simulink model "PreBraking_Scenario2_cs"  (R2014b)
settings: Solver=ode5  SolverMode=SingleTasking  StartTime=0.0  StopTime=inf  FixedStep=1/100  RelTol=1e-3
PreLoadFcn:
  | mbxruntime.callbacks.PreLoadFcn(bdroot);
  | check_NUTS_defined;
  | 
  | assignin('base',['model_closed_' bdroot],false);addpath('../includes_AEBS');
PostLoadFcn:
  | mbxruntime.callbacks.PostLoadFcn(bdroot);
InitFcn:
  | mbxruntime.callbacks.InitFcn(bdroot);
StartFcn:
  | mbxruntime.callbacks.StartFcn(bdroot);
StopFcn:
  | mbxruntime.callbacks.StopFcn(bdroot);
model workspace: external: MAT-File .\PreBraking_Scenario2_cs_hws.mat (data not in the file)
undefined symbols (not defined in the file or in its folder): mbxruntime, OrientationPitch, OrientationRoll, PositionX, PositionY, PositionZ, tabledata, warningInitialVelocity, x0
undefined symbols (not defined in the file): PreBraking_Scenario2_cs_03ca8bbbeab2b9b9, PreBraking_Scenario2_cs_060f8d532884bc4b, PreBraking_Scenario2_cs_06c37d8c8719462d, PreBraking_Scenario2_cs_0d3de4e10595602b, PreBraking_Scenario2_cs_132afc293d4bc970, PreBraking_Scenario2_cs_135fb3525bf57813, PreBraking_Scenario2_cs_199db523920b0ae8, PreBraking_Scenario2_cs_19b5c7fc995ca371, PreBraking_Scenario2_cs_1c0d05c0e95fb3bc, PreBraking_Scenario2_cs_230ed70c3742a1eb, PreBraking_Scenario2_cs_2a9a795ed7b4eca0, PreBraking_Scenario2_cs_2aad3e26cef81116, PreBraking_Scenario2_cs_3112792458948f16, PreBraking_Scenario2_cs_31511e5cf664957f, PreBraking_Scenario2_cs_335bc07f9f9d6bb2, PreBraking_Scenario2_cs_343e102d67d9e47c, PreBraking_Scenario2_cs_38754ff77a13247b, PreBraking_Scenario2_cs_3f42c52076d9af39, PreBraking_Scenario2_cs_4b3e07bd10cdcbdf, PreBraking_Scenario2_cs_4d97be448e41c5e7, PreBraking_Scenario2_cs_50fbc7e9b9a11bbd, PreBraking_Scenario2_cs_54739860340bd271, PreBraking_Scenario2_cs_5a356ab1c62c8f7e, PreBraking_Scenario2_cs_5b4437f6719e0d1b, PreBraking_Scenario2_cs_5c234b912a76c6a5, PreBraking_Scenario2_cs_6168355cd5f7aa5b, PreBraking_Scenario2_cs_622a303a40218b4d, PreBraking_Scenario2_cs_647713569694f0a8, PreBraking_Scenario2_cs_69cfdaef90de11b6, PreBraking_Scenario2_cs_6af59d93ed31b258, PreBraking_Scenario2_cs_6b0b2c155afad700, PreBraking_Scenario2_cs_6b0e277e7fb709ae, PreBraking_Scenario2_cs_6cdb8944f433c9b5, PreBraking_Scenario2_cs_6e61e0d6d53946a8, PreBraking_Scenario2_cs_721bd4ea87d705e5, PreBraking_Scenario2_cs_733181add4a3a2bd, PreBraking_Scenario2_cs_7a4dfa61d77329b3, PreBraking_Scenario2_cs_7b6eba6e821515af, PreBraking_Scenario2_cs_7dfcf0aa2939e252, PreBraking_Scenario2_cs_7f39d304a27b340b, PreBraking_Scenario2_cs_8077b8dca741d53f, PreBraking_Scenario2_cs_83874eeccd6bc572, PreBraking_Scenario2_cs_8e3f6b53dcde3bb3, PreBraking_Scenario2_cs_98c5cdaae36d0717, PreBraking_Scenario2_cs_98cfc98f5f5b01fc, PreBraking_Scenario2_cs_9906f28f708d2a62, PreBraking_Scenario2_cs_a13988e047af266f, PreBraking_Scenario2_cs_a8fd4bfaed66c690, PreBraking_Scenario2_cs_a93f6bf774ad8002, PreBraking_Scenario2_cs_a9ad9a9d247ad05d, PreBraking_Scenario2_cs_ab408108b3f0fc97, PreBraking_Scenario2_cs_Audi_A8_3_Dynamics_Simple_initialPitch, PreBraking_Scenario2_cs_Audi_A8_3_Dynamics_Simple_initialRoll, PreBraking_Scenario2_cs_Audi_A8_3_Dynamics_Simple_initialX, PreBraking_Scenario2_cs_Audi_A8_3_Dynamics_Simple_initialY, PreBraking_Scenario2_cs_Audi_A8_3_Dynamics_Simple_initialYaw, PreBraking_Scenario2_cs_Audi_A8_3_Dynamics_Simple_initialZ, PreBraking_Scenario2_cs_b1fc7fed98e6f1a7, PreBraking_Scenario2_cs_b75ef87da1419b4e, PreBraking_Scenario2_cs_b7a6524fab202de5 ... (+41)
libraries: simulink_extras x81, PreScanSimulinkLibrary x27, simulink x20, PreScanUsefulBlocks x2
(part 29 of 33)

== system PreBraking_Scenario2_cs/WheelL0_Citroen_C3_2/Actuator/visu_Rotate ==
  In1 : Inport
  sfun_RPYActuator : S-Function  FunctionName=sfun_RPYActuator  Parameters=SParameter1, SParameter2, SampleTime  EnableBusSupport=off  mask(Legacy Function){SFunctionSpec=void prescan_outputFcn(void ** work1,  PRESCAN_XYZ_DATA u1[1]), SParameter1=UniqueID, SParameter2=uint8([Object3DID 0]), SampleTime=TimeStep, ShowSpec=on}
      mask prompts: SParameter1 "P1:"; SParameter2 "P2:"; SampleTime "Sample time (-1 for inherited):"; ShowSpec "Display function specification"
      mask help:
      | This block allows you to call the legacy functions specified by the following Legacy Code Tool definition:
      | def.SFunctionName = 'sfun_PositionActuator';
      | def.OutputFcnSpec = 'void prescan_outputFcn(void ** work1,  PRESCAN_XYZ_DATA u1[1])';
      | def.StartFcnSpec = 'void prescan_startFcn(void ** work1, uint8 p1[], double p2)';
      | def.TerminateFcnSpec = 'void prescan_terminateFcn(void ** work1)';
      | def.HeaderFiles = {'prescan_positionactuator_data.h', 'prescan_header_data.h', 'prescan_SFunLibrary.h', 'prescan_CreateLogHandler.h', 'prescan_CreateErrorHandler.h'};
      | def.SourceFiles = {'prescan_MexLogHandler.cpp', 'prescan_SimStructErrorHandler.cpp', 'prescan_ConcurrentLogHandler.cpp', 'prescan_ConcurrentErrorHandler.cpp'};
      | def.HostLibFiles = {'sensorinterfaced.lib'};
      | def.TargetLibFiles = {'sensorinterfaced.so'};
      | def.IncPaths = {'.', 'C:\prescandev\vislibrary\vis\..\pimp\include\sensors\InterfaceRTW'};
      | def.SrcPaths = {'.'};
      | def.LibPaths = {'C:\\prescandev\\vislibrary_build\lib'};
      | def.SampleTime = 'parameterized';
      mask Help: <p>This block was generated automatically by the Legacy Code Tool. For detailed help on this tool, call<a href="matlab:legacy_code('help')"> legacy_code('help')</a>.</p>
      mask Callback ShowSpec:
      | if strcmp(get_param(gcbh, 'ShowSpec'), 'on')
      |   set_param(gcbh, 'MaskDisplay', sprintf('fprintf(''%s'');', get_param(gcbh, 'SFunctionSpec')));
      | else
      |   set_param(gcbh, 'MaskDisplay', sprintf('fprintf(''%s'');', get_param(gcbh, 'FunctionName')));
      | end
      mask Display: fprintf('void prescan_outputFcn(void ** work1,  PRESCAN_RPY_DATA u1[1])');
  wires:
  In1/1 -> sfun_RPYActuator/1

== system PreBraking_Scenario2_cs/WheelL0_Citroen_C3_2/Actuator/visu_Translate ==
  In1 : Inport
  sfun_PositionActuator : S-Function  FunctionName=sfun_PositionActuator  Parameters=SParameter1, SParameter2, SampleTime  EnableBusSupport=off  mask(Legacy Function){SFunctionSpec=void prescan_outputFcn(void ** work1,  PRESCAN_XYZ_DATA u1[1]), SParameter1=uint8([Object3DID 0]), SParameter2=UniqueID, SampleTime=TimeStep, ShowSpec=on}
      mask prompts: SParameter1 "P1:"; SParameter2 "P2:"; SampleTime "Sample time (-1 for inherited):"; ShowSpec "Display function specification"
      mask help:
      | This block allows you to call the legacy functions specified by the following Legacy Code Tool definition:
      | def.SFunctionName = 'sfun_PositionActuator';
      | def.OutputFcnSpec = 'void prescan_outputFcn(void ** work1,  PRESCAN_XYZ_DATA u1[1])';
      | def.StartFcnSpec = 'void prescan_startFcn(void ** work1, uint8 p1[], double p2)';
      | def.TerminateFcnSpec = 'void prescan_terminateFcn(void ** work1)';
      | def.HeaderFiles = {'prescan_positionactuator_data.h', 'prescan_header_data.h', 'prescan_SFunLibrary.h', 'prescan_CreateLogHandler.h', 'prescan_CreateErrorHandler.h'};
      | def.SourceFiles = {'prescan_MexLogHandler.cpp', 'prescan_SimStructErrorHandler.cpp', 'prescan_ConcurrentLogHandler.cpp', 'prescan_ConcurrentErrorHandler.cpp'};
      | def.HostLibFiles = {'sensorinterfaced.lib'};
      | def.TargetLibFiles = {'sensorinterfaced.so'};
      | def.IncPaths = {'.', 'C:\prescandev\vislibrary\vis\..\pimp\include\sensors\InterfaceRTW'};
      | def.SrcPaths = {'.'};
      | def.LibPaths = {'C:\\prescandev\\vislibrary_build\lib'};
      | def.SampleTime = 'parameterized';
      mask Help: <p>This block was generated automatically by the Legacy Code Tool. For detailed help on this tool, call<a href="matlab:legacy_code('help')"> legacy_code('help')</a>.</p>
      mask Callback ShowSpec:
      | if strcmp(get_param(gcbh, 'ShowSpec'), 'on')
      |   set_param(gcbh, 'MaskDisplay', sprintf('fprintf(''%s'');', get_param(gcbh, 'SFunctionSpec')));
      | else
      |   set_param(gcbh, 'MaskDisplay', sprintf('fprintf(''%s'');', get_param(gcbh, 'FunctionName')));
      | end
      mask Display: fprintf('void prescan_outputFcn(void ** work1,  PRESCAN_XYZ_DATA u1[1])');
  wires:
  In1/1 -> sfun_PositionActuator/1

== system PreBraking_Scenario2_cs/WheelL0_Fiat_Bravo_2/Actuator/visu_Rotate ==
  In1 : Inport
  sfun_RPYActuator : S-Function  FunctionName=sfun_RPYActuator  Parameters=SParameter1, SParameter2, SampleTime  EnableBusSupport=off  mask(Legacy Function){SFunctionSpec=void prescan_outputFcn(void ** work1,  PRESCAN_XYZ_DATA u1[1]), SParameter1=UniqueID, SParameter2=uint8([Object3DID 0]), SampleTime=TimeStep, ShowSpec=on}
      mask prompts: SParameter1 "P1:"; SParameter2 "P2:"; SampleTime "Sample time (-1 for inherited):"; ShowSpec "Display function specification"
      mask help:
      | This block allows you to call the legacy functions specified by the following Legacy Code Tool definition:
      | def.SFunctionName = 'sfun_PositionActuator';
      | def.OutputFcnSpec = 'void prescan_outputFcn(void ** work1,  PRESCAN_XYZ_DATA u1[1])';
      | def.StartFcnSpec = 'void prescan_startFcn(void ** work1, uint8 p1[], double p2)';
      | def.TerminateFcnSpec = 'void prescan_terminateFcn(void ** work1)';
      | def.HeaderFiles = {'prescan_positionactuator_data.h', 'prescan_header_data.h', 'prescan_SFunLibrary.h', 'prescan_CreateLogHandler.h', 'prescan_CreateErrorHandler.h'};
      | def.SourceFiles = {'prescan_MexLogHandler.cpp', 'prescan_SimStructErrorHandler.cpp', 'prescan_ConcurrentLogHandler.cpp', 'prescan_ConcurrentErrorHandler.cpp'};
      | def.HostLibFiles = {'sensorinterfaced.lib'};
      | def.TargetLibFiles = {'sensorinterfaced.so'};
      | def.IncPaths = {'.', 'C:\prescandev\vislibrary\vis\..\pimp\include\sensors\InterfaceRTW'};
      | def.SrcPaths = {'.'};
      | def.LibPaths = {'C:\\prescandev\\vislibrary_build\lib'};
      | def.SampleTime = 'parameterized';
      mask Help: <p>This block was generated automatically by the Legacy Code Tool. For detailed help on this tool, call<a href="matlab:legacy_code('help')"> legacy_code('help')</a>.</p>
      mask Callback ShowSpec:
      | if strcmp(get_param(gcbh, 'ShowSpec'), 'on')
      |   set_param(gcbh, 'MaskDisplay', sprintf('fprintf(''%s'');', get_param(gcbh, 'SFunctionSpec')));
      | else
      |   set_param(gcbh, 'MaskDisplay', sprintf('fprintf(''%s'');', get_param(gcbh, 'FunctionName')));
      | end
      mask Display: fprintf('void prescan_outputFcn(void ** work1,  PRESCAN_RPY_DATA u1[1])');
  wires:
  In1/1 -> sfun_RPYActuator/1

== system PreBraking_Scenario2_cs/WheelL0_Fiat_Bravo_2/Actuator/visu_Translate ==
  In1 : Inport
  sfun_PositionActuator : S-Function  FunctionName=sfun_PositionActuator  Parameters=SParameter1, SParameter2, SampleTime  EnableBusSupport=off  mask(Legacy Function){SFunctionSpec=void prescan_outputFcn(void ** work1,  PRESCAN_XYZ_DATA u1[1]), SParameter1=uint8([Object3DID 0]), SParameter2=UniqueID, SampleTime=TimeStep, ShowSpec=on}
      mask prompts: SParameter1 "P1:"; SParameter2 "P2:"; SampleTime "Sample time (-1 for inherited):"; ShowSpec "Display function specification"
      mask help:
      | This block allows you to call the legacy functions specified by the following Legacy Code Tool definition:
      | def.SFunctionName = 'sfun_PositionActuator';
      | def.OutputFcnSpec = 'void prescan_outputFcn(void ** work1,  PRESCAN_XYZ_DATA u1[1])';
      | def.StartFcnSpec = 'void prescan_startFcn(void ** work1, uint8 p1[], double p2)';
      | def.TerminateFcnSpec = 'void prescan_terminateFcn(void ** work1)';
      | def.HeaderFiles = {'prescan_positionactuator_data.h', 'prescan_header_data.h', 'prescan_SFunLibrary.h', 'prescan_CreateLogHandler.h', 'prescan_CreateErrorHandler.h'};
      | def.SourceFiles = {'prescan_MexLogHandler.cpp', 'prescan_SimStructErrorHandler.cpp', 'prescan_ConcurrentLogHandler.cpp', 'prescan_ConcurrentErrorHandler.cpp'};
      | def.HostLibFiles = {'sensorinterfaced.lib'};
      | def.TargetLibFiles = {'sensorinterfaced.so'};
      | def.IncPaths = {'.', 'C:\prescandev\vislibrary\vis\..\pimp\include\sensors\InterfaceRTW'};
      | def.SrcPaths = {'.'};
      | def.LibPaths = {'C:\\prescandev\\vislibrary_build\lib'};
      | def.SampleTime = 'parameterized';
      mask Help: <p>This block was generated automatically by the Legacy Code Tool. For detailed help on this tool, call<a href="matlab:legacy_code('help')"> legacy_code('help')</a>.</p>
      mask Callback ShowSpec:
      | if strcmp(get_param(gcbh, 'ShowSpec'), 'on')
      |   set_param(gcbh, 'MaskDisplay', sprintf('fprintf(''%s'');', get_param(gcbh, 'SFunctionSpec')));
      | else
      |   set_param(gcbh, 'MaskDisplay', sprintf('fprintf(''%s'');', get_param(gcbh, 'FunctionName')));
      | end
      mask Display: fprintf('void prescan_outputFcn(void ** work1,  PRESCAN_XYZ_DATA u1[1])');
  wires:
  In1/1 -> sfun_PositionActuator/1

== system PreBraking_Scenario2_cs/WheelL0_Ford_Fiesta_2/Actuator/visu_Rotate ==
  In1 : Inport
  sfun_RPYActuator : S-Function  FunctionName=sfun_RPYActuator  Parameters=SParameter1, SParameter2, SampleTime  EnableBusSupport=off  mask(Legacy Function){SFunctionSpec=void prescan_outputFcn(void ** work1,  PRESCAN_XYZ_DATA u1[1]), SParameter1=UniqueID, SParameter2=uint8([Object3DID 0]), SampleTime=TimeStep, ShowSpec=on}
      mask prompts: SParameter1 "P1:"; SParameter2 "P2:"; SampleTime "Sample time (-1 for inherited):"; ShowSpec "Display function specification"
      mask help:
      | This block allows you to call the legacy functions specified by the following Legacy Code Tool definition:
      | def.SFunctionName = 'sfun_PositionActuator';
      | def.OutputFcnSpec = 'void prescan_outputFcn(void ** work1,  PRESCAN_XYZ_DATA u1[1])';
      | def.StartFcnSpec = 'void prescan_startFcn(void ** work1, uint8 p1[], double p2)';
      | def.TerminateFcnSpec = 'void prescan_terminateFcn(void ** work1)';
      | def.HeaderFiles = {'prescan_positionactuator_data.h', 'prescan_header_data.h', 'prescan_SFunLibrary.h', 'prescan_CreateLogHandler.h', 'prescan_CreateErrorHandler.h'};
      | def.SourceFiles = {'prescan_MexLogHandler.cpp', 'prescan_SimStructErrorHandler.cpp', 'prescan_ConcurrentLogHandler.cpp', 'prescan_ConcurrentErrorHandler.cpp'};
      | def.HostLibFiles = {'sensorinterfaced.lib'};
      | def.TargetLibFiles = {'sensorinterfaced.so'};
      | def.IncPaths = {'.', 'C:\prescandev\vislibrary\vis\..\pimp\include\sensors\InterfaceRTW'};
      | def.SrcPaths = {'.'};
      | def.LibPaths = {'C:\\prescandev\\vislibrary_build\lib'};
      | def.SampleTime = 'parameterized';
      mask Help: <p>This block was generated automatically by the Legacy Code Tool. For detailed help on this tool, call<a href="matlab:legacy_code('help')"> legacy_code('help')</a>.</p>
      mask Callback ShowSpec:
      | if strcmp(get_param(gcbh, 'ShowSpec'), 'on')
      |   set_param(gcbh, 'MaskDisplay', sprintf('fprintf(''%s'');', get_param(gcbh, 'SFunctionSpec')));
      | else
      |   set_param(gcbh, 'MaskDisplay', sprintf('fprintf(''%s'');', get_param(gcbh, 'FunctionName')));
      | end
      mask Display: fprintf('void prescan_outputFcn(void ** work1,  PRESCAN_RPY_DATA u1[1])');
  wires:
  In1/1 -> sfun_RPYActuator/1

== system PreBraking_Scenario2_cs/WheelL0_Ford_Fiesta_2/Actuator/visu_Translate ==
  In1 : Inport
  sfun_PositionActuator : S-Function  FunctionName=sfun_PositionActuator  Parameters=SParameter1, SParameter2, SampleTime  EnableBusSupport=off  mask(Legacy Function){SFunctionSpec=void prescan_outputFcn(void ** work1,  PRESCAN_XYZ_DATA u1[1]), SParameter1=uint8([Object3DID 0]), SParameter2=UniqueID, SampleTime=TimeStep, ShowSpec=on}
      mask prompts: SParameter1 "P1:"; SParameter2 "P2:"; SampleTime "Sample time (-1 for inherited):"; ShowSpec "Display function specification"
      mask help:
      | This block allows you to call the legacy functions specified by the following Legacy Code Tool definition:
      | def.SFunctionName = 'sfun_PositionActuator';
      | def.OutputFcnSpec = 'void prescan_outputFcn(void ** work1,  PRESCAN_XYZ_DATA u1[1])';
      | def.StartFcnSpec = 'void prescan_startFcn(void ** work1, uint8 p1[], double p2)';
      | def.TerminateFcnSpec = 'void prescan_terminateFcn(void ** work1)';
      | def.HeaderFiles = {'prescan_positionactuator_data.h', 'prescan_header_data.h', 'prescan_SFunLibrary.h', 'prescan_CreateLogHandler.h', 'prescan_CreateErrorHandler.h'};
      | def.SourceFiles = {'prescan_MexLogHandler.cpp', 'prescan_SimStructErrorHandler.cpp', 'prescan_ConcurrentLogHandler.cpp', 'prescan_ConcurrentErrorHandler.cpp'};
      | def.HostLibFiles = {'sensorinterfaced.lib'};
      | def.TargetLibFiles = {'sensorinterfaced.so'};
      | def.IncPaths = {'.', 'C:\prescandev\vislibrary\vis\..\pimp\include\sensors\InterfaceRTW'};
      | def.SrcPaths = {'.'};
      | def.LibPaths = {'C:\\prescandev\\vislibrary_build\lib'};
      | def.SampleTime = 'parameterized';
      mask Help: <p>This block was generated automatically by the Legacy Code Tool. For detailed help on this tool, call<a href="matlab:legacy_code('help')"> legacy_code('help')</a>.</p>
      mask Callback ShowSpec:
      | if strcmp(get_param(gcbh, 'ShowSpec'), 'on')
      |   set_param(gcbh, 'MaskDisplay', sprintf('fprintf(''%s'');', get_param(gcbh, 'SFunctionSpec')));
      | else
      |   set_param(gcbh, 'MaskDisplay', sprintf('fprintf(''%s'');', get_param(gcbh, 'FunctionName')));
      | end
      mask Display: fprintf('void prescan_outputFcn(void ** work1,  PRESCAN_XYZ_DATA u1[1])');
  wires:
  In1/1 -> sfun_PositionActuator/1

== system PreBraking_Scenario2_cs/WheelL0_Toyota_Previa_2/Actuator/visu_Rotate ==
  In1 : Inport
  sfun_RPYActuator : S-Function  FunctionName=sfun_RPYActuator  Parameters=SParameter1, SParameter2, SampleTime  EnableBusSupport=off  mask(Legacy Function){SFunctionSpec=void prescan_outputFcn(void ** work1,  PRESCAN_XYZ_DATA u1[1]), SParameter1=UniqueID, SParameter2=uint8([Object3DID 0]), SampleTime=TimeStep, ShowSpec=on}
      mask prompts: SParameter1 "P1:"; SParameter2 "P2:"; SampleTime "Sample time (-1 for inherited):"; ShowSpec "Display function specification"
      mask help:
      | This block allows you to call the legacy functions specified by the following Legacy Code Tool definition:
      | def.SFunctionName = 'sfun_PositionActuator';
      | def.OutputFcnSpec = 'void prescan_outputFcn(void ** work1,  PRESCAN_XYZ_DATA u1[1])';
      | def.StartFcnSpec = 'void prescan_startFcn(void ** work1, uint8 p1[], double p2)';
      | def.TerminateFcnSpec = 'void prescan_terminateFcn(void ** work1)';
      | def.HeaderFiles = {'prescan_positionactuator_data.h', 'prescan_header_data.h', 'prescan_SFunLibrary.h', 'prescan_CreateLogHandler.h', 'prescan_CreateErrorHandler.h'};
      | def.SourceFiles = {'prescan_MexLogHandler.cpp', 'prescan_SimStructErrorHandler.cpp', 'prescan_ConcurrentLogHandler.cpp', 'prescan_ConcurrentErrorHandler.cpp'};
      | def.HostLibFiles = {'sensorinterfaced.lib'};
      | def.TargetLibFiles = {'sensorinterfaced.so'};
      | def.IncPaths = {'.', 'C:\prescandev\vislibrary\vis\..\pimp\include\sensors\InterfaceRTW'};
      | def.SrcPaths = {'.'};
      | def.LibPaths = {'C:\\prescandev\\vislibrary_build\lib'};
      | def.SampleTime = 'parameterized';
      mask Help: <p>This block was generated automatically by the Legacy Code Tool. For detailed help on this tool, call<a href="matlab:legacy_code('help')"> legacy_code('help')</a>.</p>
      mask Callback ShowSpec:
      | if strcmp(get_param(gcbh, 'ShowSpec'), 'on')
      |   set_param(gcbh, 'MaskDisplay', sprintf('fprintf(''%s'');', get_param(gcbh, 'SFunctionSpec')));
      | else
      |   set_param(gcbh, 'MaskDisplay', sprintf('fprintf(''%s'');', get_param(gcbh, 'FunctionName')));
      | end
      mask Display: fprintf('void prescan_outputFcn(void ** work1,  PRESCAN_RPY_DATA u1[1])');
  wires:
  In1/1 -> sfun_RPYActuator/1

== system PreBraking_Scenario2_cs/WheelL0_Toyota_Previa_2/Actuator/visu_Translate ==
  In1 : Inport
  sfun_PositionActuator : S-Function  FunctionName=sfun_PositionActuator  Parameters=SParameter1, SParameter2, SampleTime  EnableBusSupport=off  mask(Legacy Function){SFunctionSpec=void prescan_outputFcn(void ** work1,  PRESCAN_XYZ_DATA u1[1]), SParameter1=uint8([Object3DID 0]), SParameter2=UniqueID, SampleTime=TimeStep, ShowSpec=on}
      mask prompts: SParameter1 "P1:"; SParameter2 "P2:"; SampleTime "Sample time (-1 for inherited):"; ShowSpec "Display function specification"
      mask help:
      | This block allows you to call the legacy functions specified by the following Legacy Code Tool definition:
      | def.SFunctionName = 'sfun_PositionActuator';
      | def.OutputFcnSpec = 'void prescan_outputFcn(void ** work1,  PRESCAN_XYZ_DATA u1[1])';
      | def.StartFcnSpec = 'void prescan_startFcn(void ** work1, uint8 p1[], double p2)';
      | def.TerminateFcnSpec = 'void prescan_terminateFcn(void ** work1)';
      | def.HeaderFiles = {'prescan_positionactuator_data.h', 'prescan_header_data.h', 'prescan_SFunLibrary.h', 'prescan_CreateLogHandler.h', 'prescan_CreateErrorHandler.h'};
      | def.SourceFiles = {'prescan_MexLogHandler.cpp', 'prescan_SimStructErrorHandler.cpp', 'prescan_ConcurrentLogHandler.cpp', 'prescan_ConcurrentErrorHandler.cpp'};
      | def.HostLibFiles = {'sensorinterfaced.lib'};
      | def.TargetLibFiles = {'sensorinterfaced.so'};
      | def.IncPaths = {'.', 'C:\prescandev\vislibrary\vis\..\pimp\include\sensors\InterfaceRTW'};
      | def.SrcPaths = {'.'};
      | def.LibPaths = {'C:\\prescandev\\vislibrary_build\lib'};
      | def.SampleTime = 'parameterized';
      mask Help: <p>This block was generated automatically by the Legacy Code Tool. For detailed help on this tool, call<a href="matlab:legacy_code('help')"> legacy_code('help')</a>.</p>
      mask Callback ShowSpec:
      | if strcmp(get_param(gcbh, 'ShowSpec'), 'on')
      |   set_param(gcbh, 'MaskDisplay', sprintf('fprintf(''%s'');', get_param(gcbh, 'SFunctionSpec')));
      | else
      |   set_param(gcbh, 'MaskDisplay', sprintf('fprintf(''%s'');', get_param(gcbh, 'FunctionName')));
      | end
      mask Display: fprintf('void prescan_outputFcn(void ** work1,  PRESCAN_XYZ_DATA u1[1])');
  wires:
  In1/1 -> sfun_PositionActuator/1

== system PreBraking_Scenario2_cs/WheelL0_Toyota_Previa_3/Actuator/visu_Rotate ==
  In1 : Inport
  sfun_RPYActuator : S-Function  FunctionName=sfun_RPYActuator  Parameters=SParameter1, SParameter2, SampleTime  EnableBusSupport=off  mask(Legacy Function){SFunctionSpec=void prescan_outputFcn(void ** work1,  PRESCAN_XYZ_DATA u1[1]), SParameter1=UniqueID, SParameter2=uint8([Object3DID 0]), SampleTime=TimeStep, ShowSpec=on}
      mask prompts: SParameter1 "P1:"; SParameter2 "P2:"; SampleTime "Sample time (-1 for inherited):"; ShowSpec "Display function specification"
      mask help:
      | This block allows you to call the legacy functions specified by the following Legacy Code Tool definition:
      | def.SFunctionName = 'sfun_PositionActuator';
      | def.OutputFcnSpec = 'void prescan_outputFcn(void ** work1,  PRESCAN_XYZ_DATA u1[1])';
      | def.StartFcnSpec = 'void prescan_startFcn(void ** work1, uint8 p1[], double p2)';
      | def.TerminateFcnSpec = 'void prescan_terminateFcn(void ** work1)';
      | def.HeaderFiles = {'prescan_positionactuator_data.h', 'prescan_header_data.h', 'prescan_SFunLibrary.h', 'prescan_CreateLogHandler.h', 'prescan_CreateErrorHandler.h'};
      | def.SourceFiles = {'prescan_MexLogHandler.cpp', 'prescan_SimStructErrorHandler.cpp', 'prescan_ConcurrentLogHandler.cpp', 'prescan_ConcurrentErrorHandler.cpp'};
      | def.HostLibFiles = {'sensorinterfaced.lib'};
      | def.TargetLibFiles = {'sensorinterfaced.so'};
      | def.IncPaths = {'.', 'C:\prescandev\vislibrary\vis\..\pimp\include\sensors\InterfaceRTW'};
      | def.SrcPaths = {'.'};
      | def.LibPaths = {'C:\\prescandev\\vislibrary_build\lib'};
      | def.SampleTime = 'parameterized';
      mask Help: <p>This block was generated automatically by the Legacy Code Tool. For detailed help on this tool, call<a href="matlab:legacy_code('help')"> legacy_code('help')</a>.</p>
      mask Callback ShowSpec:
      | if strcmp(get_param(gcbh, 'ShowSpec'), 'on')
      |   set_param(gcbh, 'MaskDisplay', sprintf('fprintf(''%s'');', get_param(gcbh, 'SFunctionSpec')));
      | else
      |   set_param(gcbh, 'MaskDisplay', sprintf('fprintf(''%s'');', get_param(gcbh, 'FunctionName')));
      | end
      mask Display: fprintf('void prescan_outputFcn(void ** work1,  PRESCAN_RPY_DATA u1[1])');
  wires:
  In1/1 -> sfun_RPYActuator/1

== system PreBraking_Scenario2_cs/WheelL0_Toyota_Previa_3/Actuator/visu_Translate ==
  In1 : Inport
  sfun_PositionActuator : S-Function  FunctionName=sfun_PositionActuator  Parameters=SParameter1, SParameter2, SampleTime  EnableBusSupport=off  mask(Legacy Function){SFunctionSpec=void prescan_outputFcn(void ** work1,  PRESCAN_XYZ_DATA u1[1]), SParameter1=uint8([Object3DID 0]), SParameter2=UniqueID, SampleTime=TimeStep, ShowSpec=on}
      mask prompts: SParameter1 "P1:"; SParameter2 "P2:"; SampleTime "Sample time (-1 for inherited):"; ShowSpec "Display function specification"
      mask help:
      | This block allows you to call the legacy functions specified by the following Legacy Code Tool definition:
      | def.SFunctionName = 'sfun_PositionActuator';
      | def.OutputFcnSpec = 'void prescan_outputFcn(void ** work1,  PRESCAN_XYZ_DATA u1[1])';
      | def.StartFcnSpec = 'void prescan_startFcn(void ** work1, uint8 p1[], double p2)';
      | def.TerminateFcnSpec = 'void prescan_terminateFcn(void ** work1)';
      | def.HeaderFiles = {'prescan_positionactuator_data.h', 'prescan_header_data.h', 'prescan_SFunLibrary.h', 'prescan_CreateLogHandler.h', 'prescan_CreateErrorHandler.h'};
      | def.SourceFiles = {'prescan_MexLogHandler.cpp', 'prescan_SimStructErrorHandler.cpp', 'prescan_ConcurrentLogHandler.cpp', 'prescan_ConcurrentErrorHandler.cpp'};
      | def.HostLibFiles = {'sensorinterfaced.lib'};
      | def.TargetLibFiles = {'sensorinterfaced.so'};
      | def.IncPaths = {'.', 'C:\prescandev\vislibrary\vis\..\pimp\include\sensors\InterfaceRTW'};
      | def.SrcPaths = {'.'};
      | def.LibPaths = {'C:\\prescandev\\vislibrary_build\lib'};
      | def.SampleTime = 'parameterized';
      mask Help: <p>This block was generated automatically by the Legacy Code Tool. For detailed help on this tool, call<a href="matlab:legacy_code('help')"> legacy_code('help')</a>.</p>
      mask Callback ShowSpec:
      | if strcmp(get_param(gcbh, 'ShowSpec'), 'on')
      |   set_param(gcbh, 'MaskDisplay', sprintf('fprintf(''%s'');', get_param(gcbh, 'SFunctionSpec')));
      | else
      |   set_param(gcbh, 'MaskDisplay', sprintf('fprintf(''%s'');', get_param(gcbh, 'FunctionName')));
      | end
      mask Display: fprintf('void prescan_outputFcn(void ** work1,  PRESCAN_XYZ_DATA u1[1])');
  wires:
  In1/1 -> sfun_PositionActuator/1

== system PreBraking_Scenario2_cs/WheelL1_Audi_A8_3/Actuator/visu_Rotate ==
  In1 : Inport
  sfun_RPYActuator : S-Function  FunctionName=sfun_RPYActuator  Parameters=SParameter1, SParameter2, SampleTime  EnableBusSupport=off  mask(Legacy Function){SFunctionSpec=void prescan_outputFcn(void ** work1,  PRESCAN_XYZ_DATA u1[1]), SParameter1=UniqueID, SParameter2=uint8([Object3DID 0]), SampleTime=TimeStep, ShowSpec=on}
      mask prompts: SParameter1 "P1:"; SParameter2 "P2:"; SampleTime "Sample time (-1 for inherited):"; ShowSpec "Display function specification"
      mask help:
      | This block allows you to call the legacy functions specified by the following Legacy Code Tool definition:
      | def.SFunctionName = 'sfun_PositionActuator';
      | def.OutputFcnSpec = 'void prescan_outputFcn(void ** work1,  PRESCAN_XYZ_DATA u1[1])';
      | def.StartFcnSpec = 'void prescan_startFcn(void ** work1, uint8 p1[], double p2)';
      | def.TerminateFcnSpec = 'void prescan_terminateFcn(void ** work1)';
      | def.HeaderFiles = {'prescan_positionactuator_data.h', 'prescan_header_data.h', 'prescan_SFunLibrary.h', 'prescan_CreateLogHandler.h', 'prescan_CreateErrorHandler.h'};
      | def.SourceFiles = {'prescan_MexLogHandler.cpp', 'prescan_SimStructErrorHandler.cpp', 'prescan_ConcurrentLogHandler.cpp', 'prescan_ConcurrentErrorHandler.cpp'};
      | def.HostLibFiles = {'sensorinterfaced.lib'};
      | def.TargetLibFiles = {'sensorinterfaced.so'};
      | def.IncPaths = {'.', 'C:\prescandev\vislibrary\vis\..\pimp\include\sensors\InterfaceRTW'};
      | def.SrcPaths = {'.'};
      | def.LibPaths = {'C:\\prescandev\\vislibrary_build\lib'};
      | def.SampleTime = 'parameterized';
      mask Help: <p>This block was generated automatically by the Legacy Code Tool. For detailed help on this tool, call<a href="matlab:legacy_code('help')"> legacy_code('help')</a>.</p>
      mask Callback ShowSpec:
      | if strcmp(get_param(gcbh, 'ShowSpec'), 'on')
      |   set_param(gcbh, 'MaskDisplay', sprintf('fprintf(''%s'');', get_param(gcbh, 'SFunctionSpec')));
      | else
      |   set_param(gcbh, 'MaskDisplay', sprintf('fprintf(''%s'');', get_param(gcbh, 'FunctionName')));
      | end
      mask Display: fprintf('void prescan_outputFcn(void ** work1,  PRESCAN_RPY_DATA u1[1])');
  wires:
  In1/1 -> sfun_RPYActuator/1

== system PreBraking_Scenario2_cs/WheelL1_Audi_A8_3/Actuator/visu_Translate ==
  In1 : Inport
  sfun_PositionActuator : S-Function  FunctionName=sfun_PositionActuator  Parameters=SParameter1, SParameter2, SampleTime  EnableBusSupport=off  mask(Legacy Function){SFunctionSpec=void prescan_outputFcn(void ** work1,  PRESCAN_XYZ_DATA u1[1]), SParameter1=uint8([Object3DID 0]), SParameter2=UniqueID, SampleTime=TimeStep, ShowSpec=on}
      mask prompts: SParameter1 "P1:"; SParameter2 "P2:"; SampleTime "Sample time (-1 for inherited):"; ShowSpec "Display function specification"
      mask help:
      | This block allows you to call the legacy functions specified by the following Legacy Code Tool definition:
      | def.SFunctionName = 'sfun_PositionActuator';
      | def.OutputFcnSpec = 'void prescan_outputFcn(void ** work1,  PRESCAN_XYZ_DATA u1[1])';
      | def.StartFcnSpec = 'void prescan_startFcn(void ** work1, uint8 p1[], double p2)';
      | def.TerminateFcnSpec = 'void prescan_terminateFcn(void ** work1)';
      | def.HeaderFiles = {'prescan_positionactuator_data.h', 'prescan_header_data.h', 'prescan_SFunLibrary.h', 'prescan_CreateLogHandler.h', 'prescan_CreateErrorHandler.h'};
      | def.SourceFiles = {'prescan_MexLogHandler.cpp', 'prescan_SimStructErrorHandler.cpp', 'prescan_ConcurrentLogHandler.cpp', 'prescan_ConcurrentErrorHandler.cpp'};
      | def.HostLibFiles = {'sensorinterfaced.lib'};
      | def.TargetLibFiles = {'sensorinterfaced.so'};
      | def.IncPaths = {'.', 'C:\prescandev\vislibrary\vis\..\pimp\include\sensors\InterfaceRTW'};
      | def.SrcPaths = {'.'};
      | def.LibPaths = {'C:\\prescandev\\vislibrary_build\lib'};
      | def.SampleTime = 'parameterized';
      mask Help: <p>This block was generated automatically by the Legacy Code Tool. For detailed help on this tool, call<a href="matlab:legacy_code('help')"> legacy_code('help')</a>.</p>
      mask Callback ShowSpec:
      | if strcmp(get_param(gcbh, 'ShowSpec'), 'on')
      |   set_param(gcbh, 'MaskDisplay', sprintf('fprintf(''%s'');', get_param(gcbh, 'SFunctionSpec')));
      | else
      |   set_param(gcbh, 'MaskDisplay', sprintf('fprintf(''%s'');', get_param(gcbh, 'FunctionName')));
      | end
      mask Display: fprintf('void prescan_outputFcn(void ** work1,  PRESCAN_XYZ_DATA u1[1])');
  wires:
  In1/1 -> sfun_PositionActuator/1

== system PreBraking_Scenario2_cs/WheelL1_BMW_X5_2/Actuator/visu_Rotate ==
  In1 : Inport
  sfun_RPYActuator : S-Function  FunctionName=sfun_RPYActuator  Parameters=SParameter1, SParameter2, SampleTime  EnableBusSupport=off  mask(Legacy Function){SFunctionSpec=void prescan_outputFcn(void ** work1,  PRESCAN_XYZ_DATA u1[1]), SParameter1=UniqueID, SParameter2=uint8([Object3DID 0]), SampleTime=TimeStep, ShowSpec=on}
      mask prompts: SParameter1 "P1:"; SParameter2 "P2:"; SampleTime "Sample time (-1 for inherited):"; ShowSpec "Display function specification"
      mask help:
      | This block allows you to call the legacy functions specified by the following Legacy Code Tool definition:
      | def.SFunctionName = 'sfun_PositionActuator';
      | def.OutputFcnSpec = 'void prescan_outputFcn(void ** work1,  PRESCAN_XYZ_DATA u1[1])';
      | def.StartFcnSpec = 'void prescan_startFcn(void ** work1, uint8 p1[], double p2)';
      | def.TerminateFcnSpec = 'void prescan_terminateFcn(void ** work1)';
      | def.HeaderFiles = {'prescan_positionactuator_data.h', 'prescan_header_data.h', 'prescan_SFunLibrary.h', 'prescan_CreateLogHandler.h', 'prescan_CreateErrorHandler.h'};
      | def.SourceFiles = {'prescan_MexLogHandler.cpp', 'prescan_SimStructErrorHandler.cpp', 'prescan_ConcurrentLogHandler.cpp', 'prescan_ConcurrentErrorHandler.cpp'};
      | def.HostLibFiles = {'sensorinterfaced.lib'};
      | def.TargetLibFiles = {'sensorinterfaced.so'};
      | def.IncPaths = {'.', 'C:\prescandev\vislibrary\vis\..\pimp\include\sensors\InterfaceRTW'};
      | def.SrcPaths = {'.'};
      | def.LibPaths = {'C:\\prescandev\\vislibrary_build\lib'};
      | def.SampleTime = 'parameterized';
      mask Help: <p>This block was generated automatically by the Legacy Code Tool. For detailed help on this tool, call<a href="matlab:legacy_code('help')"> legacy_code('help')</a>.</p>
      mask Callback ShowSpec:
      | if strcmp(get_param(gcbh, 'ShowSpec'), 'on')
      |   set_param(gcbh, 'MaskDisplay', sprintf('fprintf(''%s'');', get_param(gcbh, 'SFunctionSpec')));
      | else
      |   set_param(gcbh, 'MaskDisplay', sprintf('fprintf(''%s'');', get_param(gcbh, 'FunctionName')));
      | end
      mask Display: fprintf('void prescan_outputFcn(void ** work1,  PRESCAN_RPY_DATA u1[1])');
  wires:
  In1/1 -> sfun_RPYActuator/1

== system PreBraking_Scenario2_cs/WheelL1_BMW_X5_2/Actuator/visu_Translate ==
  In1 : Inport
  sfun_PositionActuator : S-Function  FunctionName=sfun_PositionActuator  Parameters=SParameter1, SParameter2, SampleTime  EnableBusSupport=off  mask(Legacy Function){SFunctionSpec=void prescan_outputFcn(void ** work1,  PRESCAN_XYZ_DATA u1[1]), SParameter1=uint8([Object3DID 0]), SParameter2=UniqueID, SampleTime=TimeStep, ShowSpec=on}
      mask prompts: SParameter1 "P1:"; SParameter2 "P2:"; SampleTime "Sample time (-1 for inherited):"; ShowSpec "Display function specification"
      mask help:
      | This block allows you to call the legacy functions specified by the following Legacy Code Tool definition:
      | def.SFunctionName = 'sfun_PositionActuator';
      | def.OutputFcnSpec = 'void prescan_outputFcn(void ** work1,  PRESCAN_XYZ_DATA u1[1])';
      | def.StartFcnSpec = 'void prescan_startFcn(void ** work1, uint8 p1[], double p2)';
      | def.TerminateFcnSpec = 'void prescan_terminateFcn(void ** work1)';
      | def.HeaderFiles = {'prescan_positionactuator_data.h', 'prescan_header_data.h', 'prescan_SFunLibrary.h', 'prescan_CreateLogHandler.h', 'prescan_CreateErrorHandler.h'};
      | def.SourceFiles = {'prescan_MexLogHandler.cpp', 'prescan_SimStructErrorHandler.cpp', 'prescan_ConcurrentLogHandler.cpp', 'prescan_ConcurrentErrorHandler.cpp'};
      | def.HostLibFiles = {'sensorinterfaced.lib'};
      | def.TargetLibFiles = {'sensorinterfaced.so'};
      | def.IncPaths = {'.', 'C:\prescandev\vislibrary\vis\..\pimp\include\sensors\InterfaceRTW'};
      | def.SrcPaths = {'.'};
      | def.LibPaths = {'C:\\prescandev\\vislibrary_build\lib'};
      | def.SampleTime = 'parameterized';
      mask Help: <p>This block was generated automatically by the Legacy Code Tool. For detailed help on this tool, call<a href="matlab:legacy_code('help')"> legacy_code('help')</a>.</p>
      mask Callback ShowSpec:
      | if strcmp(get_param(gcbh, 'ShowSpec'), 'on')
      |   set_param(gcbh, 'MaskDisplay', sprintf('fprintf(''%s'');', get_param(gcbh, 'SFunctionSpec')));
      | else
      |   set_param(gcbh, 'MaskDisplay', sprintf('fprintf(''%s'');', get_param(gcbh, 'FunctionName')));
      | end
      mask Display: fprintf('void prescan_outputFcn(void ** work1,  PRESCAN_XYZ_DATA u1[1])');
  wires:
  In1/1 -> sfun_PositionActuator/1

== system PreBraking_Scenario2_cs/WheelL1_BMW_X5_3/Actuator/visu_Rotate ==
  In1 : Inport
  sfun_RPYActuator : S-Function  FunctionName=sfun_RPYActuator  Parameters=SParameter1, SParameter2, SampleTime  EnableBusSupport=off  mask(Legacy Function){SFunctionSpec=void prescan_outputFcn(void ** work1,  PRESCAN_XYZ_DATA u1[1]), SParameter1=UniqueID, SParameter2=uint8([Object3DID 0]), SampleTime=TimeStep, ShowSpec=on}
      mask prompts: SParameter1 "P1:"; SParameter2 "P2:"; SampleTime "Sample time (-1 for inherited):"; ShowSpec "Display function specification"
      mask help:
      | This block allows you to call the legacy functions specified by the following Legacy Code Tool definition:
      | def.SFunctionName = 'sfun_PositionActuator';
      | def.OutputFcnSpec = 'void prescan_outputFcn(void ** work1,  PRESCAN_XYZ_DATA u1[1])';
      | def.StartFcnSpec = 'void prescan_startFcn(void ** work1, uint8 p1[], double p2)';
      | def.TerminateFcnSpec = 'void prescan_terminateFcn(void ** work1)';
      | def.HeaderFiles = {'prescan_positionactuator_data.h', 'prescan_header_data.h', 'prescan_SFunLibrary.h', 'prescan_CreateLogHandler.h', 'prescan_CreateErrorHandler.h'};
      | def.SourceFiles = {'prescan_MexLogHandler.cpp', 'prescan_SimStructErrorHandler.cpp', 'prescan_ConcurrentLogHandler.cpp', 'prescan_ConcurrentErrorHandler.cpp'};
      | def.HostLibFiles = {'sensorinterfaced.lib'};
      | def.TargetLibFiles = {'sensorinterfaced.so'};
      | def.IncPaths = {'.', 'C:\prescandev\vislibrary\vis\..\pimp\include\sensors\InterfaceRTW'};
      | def.SrcPaths = {'.'};
      | def.LibPaths = {'C:\\prescandev\\vislibrary_build\lib'};
      | def.SampleTime = 'parameterized';
      mask Help: <p>This block was generated automatically by the Legacy Code Tool. For detailed help on this tool, call<a href="matlab:legacy_code('help')"> legacy_code('help')</a>.</p>
      mask Callback ShowSpec:
      | if strcmp(get_param(gcbh, 'ShowSpec'), 'on')
      |   set_param(gcbh, 'MaskDisplay', sprintf('fprintf(''%s'');', get_param(gcbh, 'SFunctionSpec')));
      | else
      |   set_param(gcbh, 'MaskDisplay', sprintf('fprintf(''%s'');', get_param(gcbh, 'FunctionName')));
      | end
      mask Display: fprintf('void prescan_outputFcn(void ** work1,  PRESCAN_RPY_DATA u1[1])');
  wires:
  In1/1 -> sfun_RPYActuator/1

== system PreBraking_Scenario2_cs/WheelL1_BMW_X5_3/Actuator/visu_Translate ==
  In1 : Inport
  sfun_PositionActuator : S-Function  FunctionName=sfun_PositionActuator  Parameters=SParameter1, SParameter2, SampleTime  EnableBusSupport=off  mask(Legacy Function){SFunctionSpec=void prescan_outputFcn(void ** work1,  PRESCAN_XYZ_DATA u1[1]), SParameter1=uint8([Object3DID 0]), SParameter2=UniqueID, SampleTime=TimeStep, ShowSpec=on}
      mask prompts: SParameter1 "P1:"; SParameter2 "P2:"; SampleTime "Sample time (-1 for inherited):"; ShowSpec "Display function specification"
      mask help:
      | This block allows you to call the legacy functions specified by the following Legacy Code Tool definition:
      | def.SFunctionName = 'sfun_PositionActuator';
      | def.OutputFcnSpec = 'void prescan_outputFcn(void ** work1,  PRESCAN_XYZ_DATA u1[1])';
      | def.StartFcnSpec = 'void prescan_startFcn(void ** work1, uint8 p1[], double p2)';
      | def.TerminateFcnSpec = 'void prescan_terminateFcn(void ** work1)';
      | def.HeaderFiles = {'prescan_positionactuator_data.h', 'prescan_header_data.h', 'prescan_SFunLibrary.h', 'prescan_CreateLogHandler.h', 'prescan_CreateErrorHandler.h'};
      | def.SourceFiles = {'prescan_MexLogHandler.cpp', 'prescan_SimStructErrorHandler.cpp', 'prescan_ConcurrentLogHandler.cpp', 'prescan_ConcurrentErrorHandler.cpp'};
      | def.HostLibFiles = {'sensorinterfaced.lib'};
      | def.TargetLibFiles = {'sensorinterfaced.so'};
      | def.IncPaths = {'.', 'C:\prescandev\vislibrary\vis\..\pimp\include\sensors\InterfaceRTW'};
      | def.SrcPaths = {'.'};
      | def.LibPaths = {'C:\\prescandev\\vislibrary_build\lib'};
      | def.SampleTime = 'parameterized';
      mask Help: <p>This block was generated automatically by the Legacy Code Tool. For detailed help on this tool, call<a href="matlab:legacy_code('help')"> legacy_code('help')</a>.</p>
      mask Callback ShowSpec:
      | if strcmp(get_param(gcbh, 'ShowSpec'), 'on')
      |   set_param(gcbh, 'MaskDisplay', sprintf('fprintf(''%s'');', get_param(gcbh, 'SFunctionSpec')));
      | else
      |   set_param(gcbh, 'MaskDisplay', sprintf('fprintf(''%s'');', get_param(gcbh, 'FunctionName')));
      | end
      mask Display: fprintf('void prescan_outputFcn(void ** work1,  PRESCAN_XYZ_DATA u1[1])');
  wires:
  In1/1 -> sfun_PositionActuator/1

== system PreBraking_Scenario2_cs/WheelL1_BMW_Z3_2/Actuator/visu_Rotate ==
  In1 : Inport
  sfun_RPYActuator : S-Function  FunctionName=sfun_RPYActuator  Parameters=SParameter1, SParameter2, SampleTime  EnableBusSupport=off  mask(Legacy Function){SFunctionSpec=void prescan_outputFcn(void ** work1,  PRESCAN_XYZ_DATA u1[1]), SParameter1=UniqueID, SParameter2=uint8([Object3DID 0]), SampleTime=TimeStep, ShowSpec=on}
      mask prompts: SParameter1 "P1:"; SParameter2 "P2:"; SampleTime "Sample time (-1 for inherited):"; ShowSpec "Display function specification"
      mask help:
      | This block allows you to call the legacy functions specified by the following Legacy Code Tool definition:
      | def.SFunctionName = 'sfun_PositionActuator';
      | def.OutputFcnSpec = 'void prescan_outputFcn(void ** work1,  PRESCAN_XYZ_DATA u1[1])';
      | def.StartFcnSpec = 'void prescan_startFcn(void ** work1, uint8 p1[], double p2)';
      | def.TerminateFcnSpec = 'void prescan_terminateFcn(void ** work1)';
      | def.HeaderFiles = {'prescan_positionactuator_data.h', 'prescan_header_data.h', 'prescan_SFunLibrary.h', 'prescan_CreateLogHandler.h', 'prescan_CreateErrorHandler.h'};
      | def.SourceFiles = {'prescan_MexLogHandler.cpp', 'prescan_SimStructErrorHandler.cpp', 'prescan_ConcurrentLogHandler.cpp', 'prescan_ConcurrentErrorHandler.cpp'};
      | def.HostLibFiles = {'sensorinterfaced.lib'};
      | def.TargetLibFiles = {'sensorinterfaced.so'};
      | def.IncPaths = {'.', 'C:\prescandev\vislibrary\vis\..\pimp\include\sensors\InterfaceRTW'};
      | def.SrcPaths = {'.'};
      | def.LibPaths = {'C:\\prescandev\\vislibrary_build\lib'};
      | def.SampleTime = 'parameterized';
      mask Help: <p>This block was generated automatically by the Legacy Code Tool. For detailed help on this tool, call<a href="matlab:legacy_code('help')"> legacy_code('help')</a>.</p>
      mask Callback ShowSpec:
      | if strcmp(get_param(gcbh, 'ShowSpec'), 'on')
      |   set_param(gcbh, 'MaskDisplay', sprintf('fprintf(''%s'');', get_param(gcbh, 'SFunctionSpec')));
      | else
      |   set_param(gcbh, 'MaskDisplay', sprintf('fprintf(''%s'');', get_param(gcbh, 'FunctionName')));
      | end
      mask Display: fprintf('void prescan_outputFcn(void ** work1,  PRESCAN_RPY_DATA u1[1])');
  wires:
  In1/1 -> sfun_RPYActuator/1

== system PreBraking_Scenario2_cs/WheelL1_BMW_Z3_2/Actuator/visu_Translate ==
  In1 : Inport
  sfun_PositionActuator : S-Function  FunctionName=sfun_PositionActuator  Parameters=SParameter1, SParameter2, SampleTime  EnableBusSupport=off  mask(Legacy Function){SFunctionSpec=void prescan_outputFcn(void ** work1,  PRESCAN_XYZ_DATA u1[1]), SParameter1=uint8([Object3DID 0]), SParameter2=UniqueID, SampleTime=TimeStep, ShowSpec=on}
      mask prompts: SParameter1 "P1:"; SParameter2 "P2:"; SampleTime "Sample time (-1 for inherited):"; ShowSpec "Display function specification"
      mask help:
      | This block allows you to call the legacy functions specified by the following Legacy Code Tool definition:
      | def.SFunctionName = 'sfun_PositionActuator';
      | def.OutputFcnSpec = 'void prescan_outputFcn(void ** work1,  PRESCAN_XYZ_DATA u1[1])';
      | def.StartFcnSpec = 'void prescan_startFcn(void ** work1, uint8 p1[], double p2)';
      | def.TerminateFcnSpec = 'void prescan_terminateFcn(void ** work1)';
      | def.HeaderFiles = {'prescan_positionactuator_data.h', 'prescan_header_data.h', 'prescan_SFunLibrary.h', 'prescan_CreateLogHandler.h', 'prescan_CreateErrorHandler.h'};
      | def.SourceFiles = {'prescan_MexLogHandler.cpp', 'prescan_SimStructErrorHandler.cpp', 'prescan_ConcurrentLogHandler.cpp', 'prescan_ConcurrentErrorHandler.cpp'};
      | def.HostLibFiles = {'sensorinterfaced.lib'};
      | def.TargetLibFiles = {'sensorinterfaced.so'};
      | def.IncPaths = {'.', 'C:\prescandev\vislibrary\vis\..\pimp\include\sensors\InterfaceRTW'};
      | def.SrcPaths = {'.'};
      | def.LibPaths = {'C:\\prescandev\\vislibrary_build\lib'};
      | def.SampleTime = 'parameterized';
      mask Help: <p>This block was generated automatically by the Legacy Code Tool. For detailed help on this tool, call<a href="matlab:legacy_code('help')"> legacy_code('help')</a>.</p>
      mask Callback ShowSpec:
      | if strcmp(get_param(gcbh, 'ShowSpec'), 'on')
      |   set_param(gcbh, 'MaskDisplay', sprintf('fprintf(''%s'');', get_param(gcbh, 'SFunctionSpec')));
      | else
      |   set_param(gcbh, 'MaskDisplay', sprintf('fprintf(''%s'');', get_param(gcbh, 'FunctionName')));
      | end
      mask Display: fprintf('void prescan_outputFcn(void ** work1,  PRESCAN_XYZ_DATA u1[1])');
  wires:
  In1/1 -> sfun_PositionActuator/1

== system PreBraking_Scenario2_cs/WheelL1_Citroen_C3_2/Actuator/visu_Rotate ==
  In1 : Inport
  sfun_RPYActuator : S-Function  FunctionName=sfun_RPYActuator  Parameters=SParameter1, SParameter2, SampleTime  EnableBusSupport=off  mask(Legacy Function){SFunctionSpec=void prescan_outputFcn(void ** work1,  PRESCAN_XYZ_DATA u1[1]), SParameter1=UniqueID, SParameter2=uint8([Object3DID 0]), SampleTime=TimeStep, ShowSpec=on}
      mask prompts: SParameter1 "P1:"; SParameter2 "P2:"; SampleTime "Sample time (-1 for inherited):"; ShowSpec "Display function specification"
      mask help:
      | This block allows you to call the legacy functions specified by the following Legacy Code Tool definition:
      | def.SFunctionName = 'sfun_PositionActuator';
      | def.OutputFcnSpec = 'void prescan_outputFcn(void ** work1,  PRESCAN_XYZ_DATA u1[1])';
      | def.StartFcnSpec = 'void prescan_startFcn(void ** work1, uint8 p1[], double p2)';
      | def.TerminateFcnSpec = 'void prescan_terminateFcn(void ** work1)';
      | def.HeaderFiles = {'prescan_positionactuator_data.h', 'prescan_header_data.h', 'prescan_SFunLibrary.h', 'prescan_CreateLogHandler.h', 'prescan_CreateErrorHandler.h'};
      | def.SourceFiles = {'prescan_MexLogHandler.cpp', 'prescan_SimStructErrorHandler.cpp', 'prescan_ConcurrentLogHandler.cpp', 'prescan_ConcurrentErrorHandler.cpp'};
      | def.HostLibFiles = {'sensorinterfaced.lib'};
      | def.TargetLibFiles = {'sensorinterfaced.so'};
      | def.IncPaths = {'.', 'C:\prescandev\vislibrary\vis\..\pimp\include\sensors\InterfaceRTW'};
      | def.SrcPaths = {'.'};
      | def.LibPaths = {'C:\\prescandev\\vislibrary_build\lib'};
      | def.SampleTime = 'parameterized';
      mask Help: <p>This block was generated automatically by the Legacy Code Tool. For detailed help on this tool, call<a href="matlab:legacy_code('help')"> legacy_code('help')</a>.</p>
      mask Callback ShowSpec:
      | if strcmp(get_param(gcbh, 'ShowSpec'), 'on')
      |   set_param(gcbh, 'MaskDisplay', sprintf('fprintf(''%s'');', get_param(gcbh, 'SFunctionSpec')));
      | else
      |   set_param(gcbh, 'MaskDisplay', sprintf('fprintf(''%s'');', get_param(gcbh, 'FunctionName')));
      | end
      mask Display: fprintf('void prescan_outputFcn(void ** work1,  PRESCAN_RPY_DATA u1[1])');
  wires:
  In1/1 -> sfun_RPYActuator/1

== system PreBraking_Scenario2_cs/WheelL1_Citroen_C3_2/Actuator/visu_Translate ==
  In1 : Inport
  sfun_PositionActuator : S-Function  FunctionName=sfun_PositionActuator  Parameters=SParameter1, SParameter2, SampleTime  EnableBusSupport=off  mask(Legacy Function){SFunctionSpec=void prescan_outputFcn(void ** work1,  PRESCAN_XYZ_DATA u1[1]), SParameter1=uint8([Object3DID 0]), SParameter2=UniqueID, SampleTime=TimeStep, ShowSpec=on}
      mask prompts: SParameter1 "P1:"; SParameter2 "P2:"; SampleTime "Sample time (-1 for inherited):"; ShowSpec "Display function specification"
      mask help:
      | This block allows you to call the legacy functions specified by the following Legacy Code Tool definition:
      | def.SFunctionName = 'sfun_PositionActuator';
      | def.OutputFcnSpec = 'void prescan_outputFcn(void ** work1,  PRESCAN_XYZ_DATA u1[1])';
      | def.StartFcnSpec = 'void prescan_startFcn(void ** work1, uint8 p1[], double p2)';
      | def.TerminateFcnSpec = 'void prescan_terminateFcn(void ** work1)';
      | def.HeaderFiles = {'prescan_positionactuator_data.h', 'prescan_header_data.h', 'prescan_SFunLibrary.h', 'prescan_CreateLogHandler.h', 'prescan_CreateErrorHandler.h'};
      | def.SourceFiles = {'prescan_MexLogHandler.cpp', 'prescan_SimStructErrorHandler.cpp', 'prescan_ConcurrentLogHandler.cpp', 'prescan_ConcurrentErrorHandler.cpp'};
      | def.HostLibFiles = {'sensorinterfaced.lib'};
      | def.TargetLibFiles = {'sensorinterfaced.so'};
      | def.IncPaths = {'.', 'C:\prescandev\vislibrary\vis\..\pimp\include\sensors\InterfaceRTW'};
      | def.SrcPaths = {'.'};
      | def.LibPaths = {'C:\\prescandev\\vislibrary_build\lib'};
      | def.SampleTime = 'parameterized';
      mask Help: <p>This block was generated automatically by the Legacy Code Tool. For detailed help on this tool, call<a href="matlab:legacy_code('help')"> legacy_code('help')</a>.</p>
      mask Callback ShowSpec:
      | if strcmp(get_param(gcbh, 'ShowSpec'), 'on')
      |   set_param(gcbh, 'MaskDisplay', sprintf('fprintf(''%s'');', get_param(gcbh, 'SFunctionSpec')));
      | else
      |   set_param(gcbh, 'MaskDisplay', sprintf('fprintf(''%s'');', get_param(gcbh, 'FunctionName')));
      | end
      mask Display: fprintf('void prescan_outputFcn(void ** work1,  PRESCAN_XYZ_DATA u1[1])');
  wires:
  In1/1 -> sfun_PositionActuator/1
